simulink model "memristors_LSTM"  (R2020b)
settings: Solver=VariableStepAuto  StartTime=0.0  StopTime=3  RelTol=1e-3
libraries: simulink x17
(part 3 of 5)

== system memristors_LSTM/Subsystem/Memristor crossbar2/Subsystem2 ==
  note: Memristor
  note: k
  note: for I-V
  note: Rmem
  note: f(x)
  note: for x
  note: for processing
  In1 : Inport
  " V" : Sin  Frequency=0.5  SampleTime=0
  2p : Gain  Gain=2
  2x : Gain  Gain=2
  Add : Sum  Inputs=-+
  Add1 : Sum
  Add2 : Sum  Inputs=-+
  Add3 : Sum  Inputs=+-
  Add4 : Sum
  Constant : Constant
  Constant10 : Constant  Value=0
  Constant4 : Constant
  Constant9 : Constant
  D : Constant  Value=10^(-8)
  Divide : Product  Inputs=*/
  Divide1 : Product  Inputs=**/
  Gain2 : Gain  Gain=0.5
  I-t : Scope
  Integrator : Integrator
  Integrator Initial condition source : Integrator  InitialConditionSource=external
  Math Function : Math  Operator=pow  SaturateOnIntegerOverflow=on
  Math Function1 : Math  Operator=square  SaturateOnIntegerOverflow=on
  Product1 : Product
  Product2 : Product
  Product3 : Product  Inputs=3
  Product4 : Product
  R_off : Constant  Value=20000
  R_on : Constant  Value=100
  R_on1 : Constant  Value=100
  Switch : Switch  Threshold=1
  Switch1 : Switch
  V-t : Scope
  p : Constant  Value=10
  x-t : Scope
  x0 : Constant  Value=0.7
  𝜇_𝑣 : Constant  Value=10^(-14)
  Out1 : Outport
  Out2 : Outport  Port=2
  wires:
  Constant9/1 -> Switch/1
  Switch/1 -> Switch1/2, Switch1/1
  R_on/1 -> Divide1/1
  Integrator Initial condition source/1 -> Switch/3, Switch/2, x-t/1
  2p/1 -> Math Function/2
  Divide/1 -> I-t/1, Product3/1
  Switch1/1 -> Product2/2, Add/1, 2x/1
  𝜇_𝑣/1 -> Divide1/2
  Gain2/1 -> Integrator/1
  Math Function/1 -> Add3/2
  Add/1 -> Product1/1
  R_on1/1 -> Product2/1
  Constant/1 -> Add/2
  p/1 -> 2p/1
  D/1 -> Math Function1/1
  Divide1/1 -> Product3/3
  2x/1 -> Add2/2
  Product1/1 -> Add1/2
  R_off/1 -> Product1/2
  Add2/1 -> Math Function/1
  Constant4/1 -> Add3/1, Add2/1
  Product4/1 -> Out1/1, Out2/1, V-t/1
  Product2/1 -> Add1/1
  x0/1 -> Integrator Initial condition source/2
  Constant10/1 -> Switch1/3
  Product3/1 -> Integrator Initial condition source/1
  Add1/1 -> Divide/2
  Add3/1 -> Product3/2
  Math Function1/1 -> Divide1/3
  " V"/1 -> Add4/2
  In1/1 -> Add4/1
  Add4/1 -> Product4/1, Gain2/1
  Integrator/1 -> Divide/1, Product4/2

== system memristors_LSTM/Subsystem/Memristor crossbar2/Subsystem20 ==
  note: Memristor
  note: k
  note: for I-V
  note: Rmem
  note: f(x)
  note: for x
  note: for processing
  " V" : Sin  Amplitude=0.1  Frequency=0.5  SampleTime=0
  2p : Gain  Gain=2
  2x : Gain  Gain=2
  Add : Sum  Inputs=-+
  Add1 : Sum
  Add2 : Sum  Inputs=-+
  Add3 : Sum  Inputs=+-
  Constant : Constant
  Constant10 : Constant  Value=0
  Constant4 : Constant
  Constant9 : Constant
  D : Constant  Value=10^(-8)
  Divide : Product  Inputs=*/
  Divide1 : Product  Inputs=**/
  Gain2 : Gain  Gain=0.5
  I-t : Scope
  Integrator : Integrator
  Integrator Initial condition source : Integrator  InitialConditionSource=external
  Math Function : Math  Operator=pow  SaturateOnIntegerOverflow=on
  Math Function1 : Math  Operator=square  SaturateOnIntegerOverflow=on
  Product1 : Product
  Product2 : Product
  Product3 : Product  Inputs=3
  Product4 : Product
  R_off : Constant  Value=20000
  R_on : Constant  Value=100
  R_on1 : Constant  Value=100
  Switch : Switch  Threshold=1
  Switch1 : Switch
  V-t : Scope
  p : Constant  Value=10
  x-t : Scope
  x0 : Constant  Value=0.7
  𝜇_𝑣 : Constant  Value=10^(-14)
  Out1 : Outport
  Out2 : Outport  Port=2
  wires:
  Constant9/1 -> Switch/1
  Switch/1 -> Switch1/2, Switch1/1
  R_on/1 -> Divide1/1
  Integrator Initial condition source/1 -> Switch/3, Switch/2, x-t/1
  Integrator/1 -> Divide/1, Product4/2
  2p/1 -> Math Function/2
  Divide/1 -> I-t/1, Product3/1
  Switch1/1 -> Product2/2, Add/1, 2x/1
  𝜇_𝑣/1 -> Divide1/2
  Gain2/1 -> Integrator/1
  Math Function/1 -> Add3/2
  Add/1 -> Product1/1
  R_on1/1 -> Product2/1
  Constant/1 -> Add/2
  p/1 -> 2p/1
  D/1 -> Math Function1/1
  Divide1/1 -> Product3/3
  2x/1 -> Add2/2
  Product1/1 -> Add1/2
  R_off/1 -> Product1/2
  Add2/1 -> Math Function/1
  Constant4/1 -> Add3/1, Add2/1
  Product4/1 -> Out1/1, Out2/1, V-t/1
  Product2/1 -> Add1/1
  x0/1 -> Integrator Initial condition source/2
  Constant10/1 -> Switch1/3
  Product3/1 -> Integrator Initial condition source/1
  Add1/1 -> Divide/2
  Add3/1 -> Product3/2
  Math Function1/1 -> Divide1/3
  " V"/1 -> Gain2/1, Product4/1

== system memristors_LSTM/Subsystem/Memristor crossbar2/Subsystem21 ==
  note: Memristor
  note: k
  note: for I-V
  note: Rmem
  note: f(x)
  note: for x
  note: for processing
  In1 : Inport
  " V" : Sin  Amplitude=0.1  Frequency=0.5  SampleTime=0
  2p : Gain  Gain=2
  2x : Gain  Gain=2
  Add : Sum  Inputs=-+
  Add1 : Sum
  Add2 : Sum  Inputs=-+
  Add3 : Sum  Inputs=+-
  Add4 : Sum
  Constant : Constant
  Constant10 : Constant  Value=0
  Constant4 : Constant
  Constant9 : Constant
  D : Constant  Value=10^(-8)
  Divide : Product  Inputs=*/
  Divide1 : Product  Inputs=**/
  Gain2 : Gain  Gain=0.5
  I-t : Scope
  Integrator : Integrator
  Integrator Initial condition source : Integrator  InitialConditionSource=external
  Math Function : Math  Operator=pow  SaturateOnIntegerOverflow=on
  Math Function1 : Math  Operator=square  SaturateOnIntegerOverflow=on
  Product1 : Product
  Product2 : Product
  Product3 : Product  Inputs=3
  Product4 : Product
  R_off : Constant  Value=20000
  R_on : Constant  Value=100
  R_on1 : Constant  Value=100
  Switch : Switch  Threshold=1
  Switch1 : Switch
  V-t : Scope
  p : Constant  Value=10
  x-t : Scope
  x0 : Constant  Value=0.7
  𝜇_𝑣 : Constant  Value=10^(-14)
  Out1 : Outport
  Out2 : Outport  Port=2
  wires:
  Constant9/1 -> Switch/1
  Switch/1 -> Switch1/2, Switch1/1
  R_on/1 -> Divide1/1
  Integrator Initial condition source/1 -> Switch/3, Switch/2, x-t/1
  2p/1 -> Math Function/2
  Divide/1 -> I-t/1, Product3/1
  Switch1/1 -> Product2/2, Add/1, 2x/1
  𝜇_𝑣/1 -> Divide1/2
  Gain2/1 -> Integrator/1
  Math Function/1 -> Add3/2
  Add/1 -> Product1/1
  R_on1/1 -> Product2/1
  Constant/1 -> Add/2
  p/1 -> 2p/1
  D/1 -> Math Function1/1
  Divide1/1 -> Product3/3
  2x/1 -> Add2/2
  Product1/1 -> Add1/2
  R_off/1 -> Product1/2
  Add2/1 -> Math Function/1
  Constant4/1 -> Add3/1, Add2/1
  Product4/1 -> Out1/1, Out2/1, V-t/1
  Product2/1 -> Add1/1
  x0/1 -> Integrator Initial condition source/2
  Constant10/1 -> Switch1/3
  Product3/1 -> Integrator Initial condition source/1
  Add1/1 -> Divide/2
  Add3/1 -> Product3/2
  Math Function1/1 -> Divide1/3
  " V"/1 -> Add4/2
  In1/1 -> Add4/1
  Add4/1 -> Product4/1, Gain2/1
  Integrator/1 -> Divide/1, Product4/2

== system memristors_LSTM/Subsystem/Memristor crossbar2/Subsystem22 ==
  note: k
  note: for I-V
  note: Rmem
  note: f(x)
  note: for x
  note: for processing
  In1 : Inport
  " V" : Sin  Amplitude=0.1  Frequency=0.5  SampleTime=0
  2p : Gain  Gain=2
  2x : Gain  Gain=2
  Add : Sum  Inputs=-+
  Add1 : Sum
  Add2 : Sum  Inputs=-+
  Add3 : Sum  Inputs=+-
  Add4 : Sum
  Constant : Constant
  Constant10 : Constant  Value=0
  Constant4 : Constant
  Constant9 : Constant
  D : Constant  Value=10^(-8)
  Divide : Product  Inputs=*/
  Divide1 : Product  Inputs=**/
  Gain2 : Gain  Gain=0.5
  I-t : Scope
  Integrator : Integrator
  Integrator Initial condition source : Integrator  InitialConditionSource=external
  Math Function : Math  Operator=pow  SaturateOnIntegerOverflow=on
  Math Function1 : Math  Operator=square  SaturateOnIntegerOverflow=on
  Product1 : Product
  Product2 : Product
  Product3 : Product  Inputs=3
  Product4 : Product
  R_off : Constant  Value=20000
  R_on : Constant  Value=100
  R_on1 : Constant  Value=100
  Switch : Switch  Threshold=1
  Switch1 : Switch
  V-t : Scope
  p : Constant  Value=10
  x-t : Scope
  x0 : Constant  Value=0.7
  𝜇_𝑣 : Constant  Value=10^(-14)
  Out1 : Outport
  Out2 : Outport  Port=2
  wires:
  Constant9/1 -> Switch/1
  Switch/1 -> Switch1/2, Switch1/1
  R_on/1 -> Divide1/1
  Integrator Initial condition source/1 -> Switch/3, Switch/2, x-t/1
  Integrator/1 -> Divide/1, Product4/2
  2p/1 -> Math Function/2
  Divide/1 -> I-t/1, Product3/1
  Switch1/1 -> Product2/2, Add/1, 2x/1
  𝜇_𝑣/1 -> Divide1/2
  Gain2/1 -> Integrator/1
  Math Function/1 -> Add3/2
  Add/1 -> Product1/1
  R_on1/1 -> Product2/1
  Constant/1 -> Add/2
  p/1 -> 2p/1
  D/1 -> Math Function1/1
  Divide1/1 -> Product3/3
  2x/1 -> Add2/2
  Product1/1 -> Add1/2
  R_off/1 -> Product1/2
  Add2/1 -> Math Function/1
  Constant4/1 -> Add3/1, Add2/1
  Product2/1 -> Add1/1
  x0/1 -> Integrator Initial condition source/2
  Constant10/1 -> Switch1/3
  Product3/1 -> Integrator Initial condition source/1
  Add1/1 -> Divide/2
  Add3/1 -> Product3/2
  Math Function1/1 -> Divide1/3
  " V"/1 -> Add4/2
  In1/1 -> Add4/1
  Add4/1 -> Product4/1, Gain2/1
  Product4/1 -> Out1/1, Out2/1, V-t/1

== system memristors_LSTM/Subsystem/Memristor crossbar2/Subsystem23 ==
  note: Memristor
  note: k
  note: for I-V
  note: Rmem
  note: f(x)
  note: for x
  note: for processing
  In1 : Inport
  " V" : Sin  Amplitude=0.1  Frequency=0.5  SampleTime=0
  2p : Gain  Gain=2
  2x : Gain  Gain=2
  Add : Sum  Inputs=-+
  Add1 : Sum
  Add2 : Sum  Inputs=-+
  Add3 : Sum  Inputs=+-
  Add4 : Sum
  Constant : Constant
  Constant10 : Constant  Value=0
  Constant4 : Constant
  Constant9 : Constant
  D : Constant  Value=10^(-8)
  Divide : Product  Inputs=*/
  Divide1 : Product  Inputs=**/
  Gain2 : Gain  Gain=0.5
  I-t : Scope
  Integrator : Integrator
  Integrator Initial condition source : Integrator  InitialConditionSource=external
  Math Function : Math  Operator=pow  SaturateOnIntegerOverflow=on
  Math Function1 : Math  Operator=square  SaturateOnIntegerOverflow=on
  Product1 : Product
  Product2 : Product
  Product3 : Product  Inputs=3
  Product4 : Product
  R_off : Constant  Value=20000
  R_on : Constant  Value=100
  R_on1 : Constant  Value=100
  Switch : Switch  Threshold=1
  Switch1 : Switch
  V-t : Scope
  p : Constant  Value=10
  x-t : Scope
  x0 : Constant  Value=0.7
  𝜇_𝑣 : Constant  Value=10^(-14)
  Out1 : Outport
  Out2 : Outport  Port=2
  wires:
  Constant9/1 -> Switch/1
  Switch/1 -> Switch1/2, Switch1/1
  R_on/1 -> Divide1/1
  Integrator Initial condition source/1 -> Switch/3, Switch/2, x-t/1
  Integrator/1 -> Divide/1, Product4/2
  2p/1 -> Math Function/2
  Divide/1 -> I-t/1, Product3/1
  Switch1/1 -> Product2/2, Add/1, 2x/1
  𝜇_𝑣/1 -> Divide1/2
  Gain2/1 -> Integrator/1
  Math Function/1 -> Add3/2
  Add/1 -> Product1/1
  R_on1/1 -> Product2/1
  Constant/1 -> Add/2
  p/1 -> 2p/1
  D/1 -> Math Function1/1
  Divide1/1 -> Product3/3
  2x/1 -> Add2/2
  Product1/1 -> Add1/2
  R_off/1 -> Product1/2
  Add2/1 -> Math Function/1
  Constant4/1 -> Add3/1, Add2/1
  Product4/1 -> Out1/1, Out2/1, V-t/1
  Product2/1 -> Add1/1
  x0/1 -> Integrator Initial condition source/2
  Constant10/1 -> Switch1/3
  Product3/1 -> Integrator Initial condition source/1
  Add1/1 -> Divide/2
  Add3/1 -> Product3/2
  Math Function1/1 -> Divide1/3
  " V"/1 -> Add4/2
  In1/1 -> Add4/1
  Add4/1 -> Product4/1, Gain2/1

== system memristors_LSTM/Subsystem/Memristor crossbar2/Subsystem24 ==
  note: Memristor
  note: k
  note: for I-V
  note: Rmem
  note: f(x)
  note: for x
  note: for processing
  In1 : Inport
  " V" : Sin  Amplitude=0.1  Frequency=0.5  SampleTime=0
  2p : Gain  Gain=2
  2x : Gain  Gain=2
  Add : Sum  Inputs=-+
  Add1 : Sum
  Add2 : Sum  Inputs=-+
  Add3 : Sum  Inputs=+-
  Add4 : Sum
  Constant : Constant
  Constant10 : Constant  Value=0
  Constant4 : Constant
  Constant9 : Constant
  D : Constant  Value=10^(-8)
  Divide : Product  Inputs=*/
  Divide1 : Product  Inputs=**/
  Gain2 : Gain  Gain=0.5
  I-t : Scope
  Integrator : Integrator
  Integrator Initial condition source : Integrator  InitialConditionSource=external
  Math Function : Math  Operator=pow  SaturateOnIntegerOverflow=on
  Math Function1 : Math  Operator=square  SaturateOnIntegerOverflow=on
  Product1 : Product
  Product2 : Product
  Product3 : Product  Inputs=3
  Product4 : Product
  R_off : Constant  Value=20000
  R_on : Constant  Value=100
  R_on1 : Constant  Value=100
  Switch : Switch  Threshold=1
  Switch1 : Switch
  V-t : Scope
  XY Graph : simulink/Sinks/XY Graph  xmin=-1  xmax=1  ymin=-1  ymax=1  st=-1
  p : Constant  Value=10
  x-t : Scope
  x0 : Constant  Value=0.7
  𝜇_𝑣 : Constant  Value=10^(-14)
  Out2 : Outport
  wires:
  Constant9/1 -> Switch/1
  Switch/1 -> Switch1/2, Switch1/1
  R_on/1 -> Divide1/1
  Integrator Initial condition source/1 -> Switch/3, Switch/2, x-t/1
  Integrator/1 -> Divide/1, Product4/2
  2p/1 -> Math Function/2
  Divide/1 -> XY Graph/2, I-t/1, Product3/1
  Switch1/1 -> Product2/2, Add/1, 2x/1
  𝜇_𝑣/1 -> Divide1/2
  Gain2/1 -> Integrator/1
  Math Function/1 -> Add3/2
  Add/1 -> Product1/1
  R_on1/1 -> Product2/1
  Constant/1 -> Add/2
  p/1 -> 2p/1
  D/1 -> Math Function1/1
  Divide1/1 -> Product3/3
  2x/1 -> Add2/2
  Product1/1 -> Add1/2
  R_off/1 -> Product1/2
  Add2/1 -> Math Function/1
  Constant4/1 -> Add3/1, Add2/1
  Product2/1 -> Add1/1
  x0/1 -> Integrator Initial condition source/2
  Constant10/1 -> Switch1/3
  Product3/1 -> Integrator Initial condition source/1
  Add1/1 -> Divide/2
  Add3/1 -> Product3/2
  Math Function1/1 -> Divide1/3
  " V"/1 -> Add4/2
  In1/1 -> Add4/1
  Add4/1 -> Product4/1, Gain2/1
  Product4/1 -> XY Graph/1, Out2/1, V-t/1

== system memristors_LSTM/Subsystem/Memristor crossbar2/Subsystem25 ==
  note: k
  note: for I-V
  note: Rmem
  note: f(x)
  note: for x
  note: for processing
  In1 : Inport
  " V" : Sin  Frequency=0.5  SampleTime=0
  2p : Gain  Gain=2
  2x : Gain  Gain=2
  Add : Sum  Inputs=-+
  Add1 : Sum
  Add2 : Sum  Inputs=-+
  Add3 : Sum  Inputs=+-
  Add4 : Sum
  Constant : Constant
  Constant10 : Constant  Value=0
  Constant4 : Constant
  Constant9 : Constant
  D : Constant  Value=10^(-8)
  Divide : Product  Inputs=*/
  Divide1 : Product  Inputs=**/
  Gain2 : Gain  Gain=0.5
  I-t : Scope
  Integrator : Integrator
  Integrator Initial condition source : Integrator  InitialConditionSource=external
  Math Function : Math  Operator=pow  SaturateOnIntegerOverflow=on
  Math Function1 : Math  Operator=square  SaturateOnIntegerOverflow=on
  Product1 : Product
  Product2 : Product
  Product3 : Product  Inputs=3
  Product4 : Product
  R_off : Constant  Value=20000
  R_on : Constant  Value=100
  R_on1 : Constant  Value=100
  Switch : Switch  Threshold=1
  Switch1 : Switch
  V-t : Scope
  p : Constant  Value=10
  x-t : Scope
  x0 : Constant  Value=0.7
  𝜇_𝑣 : Constant  Value=10^(-14)
  Out1 : Outport
  Out2 : Outport  Port=2
  wires:
  Constant9/1 -> Switch/1
  Switch/1 -> Switch1/2, Switch1/1
  R_on/1 -> Divide1/1
  Integrator Initial condition source/1 -> Switch/3, Switch/2, x-t/1
  Integrator/1 -> Divide/1, Product4/2
  2p/1 -> Math Function/2
  Divide/1 -> I-t/1, Product3/1
  Switch1/1 -> Product2/2, Add/1, 2x/1
  𝜇_𝑣/1 -> Divide1/2
  Gain2/1 -> Integrator/1
  Math Function/1 -> Add3/2
  Add/1 -> Product1/1
  R_on1/1 -> Product2/1
  Constant/1 -> Add/2
  p/1 -> 2p/1
  D/1 -> Math Function1/1
  Divide1/1 -> Product3/3
  2x/1 -> Add2/2
  Product1/1 -> Add1/2
  R_off/1 -> Product1/2
  Add2/1 -> Math Function/1
  Constant4/1 -> Add3/1, Add2/1
  Product2/1 -> Add1/1
  x0/1 -> Integrator Initial condition source/2
  Constant10/1 -> Switch1/3
  Product3/1 -> Integrator Initial condition source/1
  Add1/1 -> Divide/2
  Add3/1 -> Product3/2
  Math Function1/1 -> Divide1/3
  " V"/1 -> Add4/2
  In1/1 -> Add4/1
  Add4/1 -> Product4/1, Gain2/1
  Product4/1 -> Out1/1, Out2/1, V-t/1

== system memristors_LSTM/Subsystem/Memristor crossbar2/Subsystem3 ==
  note: Memristor
  note: k
  note: for I-V
  note: Rmem
  note: f(x)
  note: for x
  note: for processing
  In1 : Inport
  " V" : Sin  Frequency=0.5  SampleTime=0
  2p : Gain  Gain=2
  2x : Gain  Gain=2
  Add : Sum  Inputs=-+
  Add1 : Sum
  Add2 : Sum  Inputs=-+
  Add3 : Sum  Inputs=+-
  Add4 : Sum
  Constant : Constant
  Constant10 : Constant  Value=0
  Constant4 : Constant
  Constant9 : Constant
  D : Constant  Value=10^(-8)
  Divide : Product  Inputs=*/
  Divide1 : Product  Inputs=**/
  Gain2 : Gain  Gain=0.5
  I-t : Scope
  Integrator : Integrator
  Integrator Initial condition source : Integrator  InitialConditionSource=external
  Math Function : Math  Operator=pow  SaturateOnIntegerOverflow=on
  Math Function1 : Math  Operator=square  SaturateOnIntegerOverflow=on
  Product1 : Product
  Product2 : Product
  Product3 : Product  Inputs=3
  Product4 : Product
  R_off : Constant  Value=20000
  R_on : Constant  Value=100
  R_on1 : Constant  Value=100
  Switch : Switch  Threshold=1
  Switch1 : Switch
  V-t : Scope
  p : Constant  Value=10
  x-t : Scope
  x0 : Constant  Value=0.7
  𝜇_𝑣 : Constant  Value=10^(-14)
  Out1 : Outport
  Out2 : Outport  Port=2
  wires:
  Constant9/1 -> Switch/1
  Switch/1 -> Switch1/2, Switch1/1
  R_on/1 -> Divide1/1
  Integrator Initial condition source/1 -> Switch/3, Switch/2, x-t/1
  Integrator/1 -> Divide/1, Product4/2
  2p/1 -> Math Function/2
  Divide/1 -> I-t/1, Product3/1
  Switch1/1 -> Product2/2, Add/1, 2x/1
  𝜇_𝑣/1 -> Divide1/2
  Gain2/1 -> Integrator/1
  Math Function/1 -> Add3/2
  Add/1 -> Product1/1
  R_on1/1 -> Product2/1
  Constant/1 -> Add/2
  p/1 -> 2p/1
  D/1 -> Math Function1/1
  Divide1/1 -> Product3/3
  2x/1 -> Add2/2
  Product1/1 -> Add1/2
  R_off/1 -> Product1/2
  Add2/1 -> Math Function/1
  Constant4/1 -> Add3/1, Add2/1
  Product4/1 -> Out1/1, Out2/1, V-t/1
  Product2/1 -> Add1/1
  x0/1 -> Integrator Initial condition source/2
  Constant10/1 -> Switch1/3
  Product3/1 -> Integrator Initial condition source/1
  Add1/1 -> Divide/2
  Add3/1 -> Product3/2
  Math Function1/1 -> Divide1/3
  " V"/1 -> Add4/2
  In1/1 -> Add4/1
  Add4/1 -> Product4/1, Gain2/1

== system memristors_LSTM/Subsystem/Memristor crossbar2/Subsystem4 ==
  note: Memristor
  note: k
  note: for I-V
  note: Rmem
  note: f(x)
  note: for x
  note: for processing
  In1 : Inport
  " V" : Sin  Frequency=0.5  SampleTime=0
  2p : Gain  Gain=2
  2x : Gain  Gain=2
  Add : Sum  Inputs=-+
  Add1 : Sum
  Add2 : Sum  Inputs=-+
  Add3 : Sum  Inputs=+-
  Add4 : Sum
  Constant : Constant
  Constant10 : Constant  Value=0
  Constant4 : Constant
  Constant9 : Constant
  D : Constant  Value=10^(-8)
  Divide : Product  Inputs=*/
  Divide1 : Product  Inputs=**/
  Gain2 : Gain  Gain=0.5
  I-t : Scope
  Integrator : Integrator
  Integrator Initial condition source : Integrator  InitialConditionSource=external
  Math Function : Math  Operator=pow  SaturateOnIntegerOverflow=on
  Math Function1 : Math  Operator=square  SaturateOnIntegerOverflow=on
  Product1 : Product
  Product2 : Product
  Product3 : Product  Inputs=3
  Product4 : Product
  R_off : Constant  Value=20000
  R_on : Constant  Value=100
  R_on1 : Constant  Value=100
  Switch : Switch  Threshold=1
  Switch1 : Switch
  V-t : Scope
  p : Constant  Value=10
  x-t : Scope
  x0 : Constant  Value=0.7
  𝜇_𝑣 : Constant  Value=10^(-14)
  Out2 : Outport
  wires:
  Constant9/1 -> Switch/1
  Switch/1 -> Switch1/2, Switch1/1
  R_on/1 -> Divide1/1
  Integrator Initial condition source/1 -> Switch/3, Switch/2, x-t/1
  Integrator/1 -> Divide/1, Product4/2
  2p/1 -> Math Function/2
  Divide/1 -> I-t/1, Product3/1
  Switch1/1 -> Product2/2, Add/1, 2x/1
  𝜇_𝑣/1 -> Divide1/2
  Gain2/1 -> Integrator/1
  Math Function/1 -> Add3/2
  Add/1 -> Product1/1
  R_on1/1 -> Product2/1
  Constant/1 -> Add/2
  p/1 -> 2p/1
  D/1 -> Math Function1/1
  Divide1/1 -> Product3/3
  2x/1 -> Add2/2
  Product1/1 -> Add1/2
  R_off/1 -> Product1/2
  Add2/1 -> Math Function/1
  Constant4/1 -> Add3/1, Add2/1
  Product4/1 -> Out2/1, V-t/1
  Product2/1 -> Add1/1
  x0/1 -> Integrator Initial condition source/2
  Constant10/1 -> Switch1/3
  Product3/1 -> Integrator Initial condition source/1
  Add1/1 -> Divide/2
  Add3/1 -> Product3/2
  Math Function1/1 -> Divide1/3
  " V"/1 -> Add4/2
  In1/1 -> Add4/1
  Add4/1 -> Product4/1, Gain2/1

== system memristors_LSTM/Subsystem/Memristor crossbar2/Subsystem5 ==
  note: Memristor
  note: k
  note: for I-V
  note: Rmem
  note: f(x)
  note: for x
  note: for processing
  " V" : Sin  Amplitude=0.1  Frequency=0.5  SampleTime=0
  2p : Gain  Gain=2
  2x : Gain  Gain=2
  Add : Sum  Inputs=-+
  Add1 : Sum
  Add2 : Sum  Inputs=-+
  Add3 : Sum  Inputs=+-
  Constant : Constant
  Constant10 : Constant  Value=0
  Constant4 : Constant
  Constant9 : Constant
  D : Constant  Value=10^(-8)
  Divide : Product  Inputs=*/
  Divide1 : Product  Inputs=**/
  Gain2 : Gain  Gain=0.5
  I-t : Scope
  Integrator : Integrator
  Integrator Initial condition source : Integrator  InitialConditionSource=external
  Math Function : Math  Operator=pow  SaturateOnIntegerOverflow=on
  Math Function1 : Math  Operator=square  SaturateOnIntegerOverflow=on
  Product1 : Product
  Product2 : Product
  Product3 : Product  Inputs=3
  Product4 : Product
  R_off : Constant  Value=20000
  R_on : Constant  Value=100
  R_on1 : Constant  Value=100
  Switch : Switch  Threshold=1
  Switch1 : Switch
  V-t : Scope
  p : Constant  Value=10
  x-t : Scope
  x0 : Constant  Value=0.7
  𝜇_𝑣 : Constant  Value=10^(-14)
  Out1 : Outport
  Out2 : Outport  Port=2
  wires:
  Constant9/1 -> Switch/1
  Switch/1 -> Switch1/2, Switch1/1
  R_on/1 -> Divide1/1
  Integrator Initial condition source/1 -> Switch/3, Switch/2, x-t/1
  Integrator/1 -> Divide/1, Product4/2
  2p/1 -> Math Function/2
  Divide/1 -> I-t/1, Product3/1
  Switch1/1 -> Product2/2, Add/1, 2x/1
  𝜇_𝑣/1 -> Divide1/2
  Gain2/1 -> Integrator/1
  Math Function/1 -> Add3/2
  Add/1 -> Product1/1
  R_on1/1 -> Product2/1
  Constant/1 -> Add/2
  p/1 -> 2p/1
  D/1 -> Math Function1/1
  Divide1/1 -> Product3/3
  2x/1 -> Add2/2
  Product1/1 -> Add1/2
  R_off/1 -> Product1/2
  Add2/1 -> Math Function/1
  Constant4/1 -> Add3/1, Add2/1
  Product4/1 -> Out1/1, Out2/1, V-t/1
  Product2/1 -> Add1/1
  x0/1 -> Integrator Initial condition source/2
  Constant10/1 -> Switch1/3
  Product3/1 -> Integrator Initial condition source/1
  Add1/1 -> Divide/2
  Add3/1 -> Product3/2
  Math Function1/1 -> Divide1/3
  " V"/1 -> Gain2/1, Product4/1

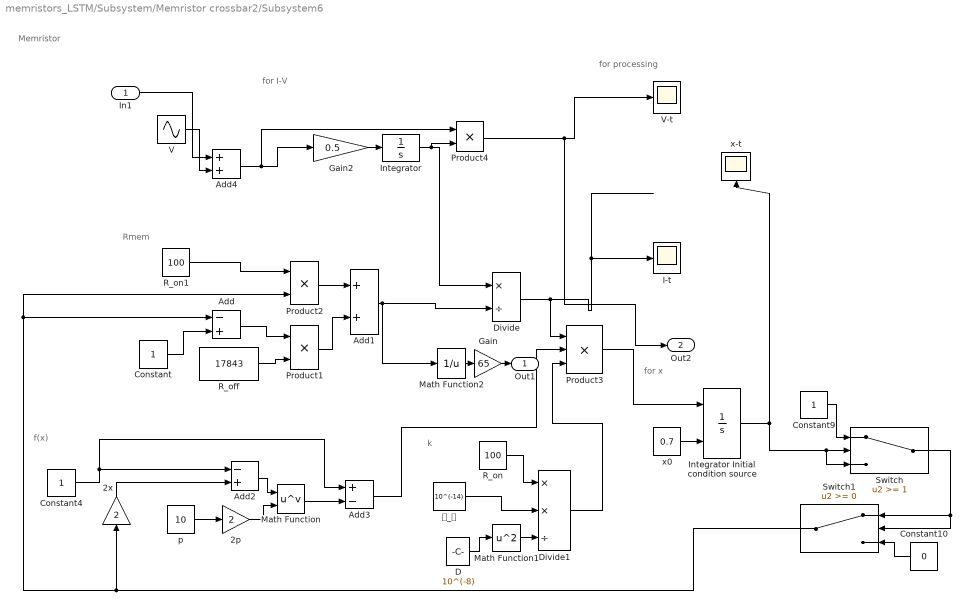
== system memristors_LSTM/Subsystem/Memristor crossbar2/Subsystem6 ==
  note: Memristor
  note: k
  note: for I-V
  note: Rmem
  note: f(x)
  note: for x
  note: for processing
  In1 : Inport
  " V" : Sin  Frequency=0.5  SampleTime=0
  2p : Gain  Gain=2
  2x : Gain  Gain=2
  Add : Sum  Inputs=-+
  Add1 : Sum
  Add2 : Sum  Inputs=-+
  Add3 : Sum  Inputs=+-
  Add4 : Sum
  Constant : Constant
  Constant10 : Constant  Value=0
  Constant4 : Constant
  Constant9 : Constant
  D : Constant  Value=10^(-8)
  Divide : Product  Inputs=*/
  Divide1 : Product  Inputs=**/
  Gain : Gain  Gain=65
  Gain2 : Gain  Gain=0.5
  I-t : Scope
  Integrator : Integrator
  Integrator Initial condition source : Integrator  InitialConditionSource=external
  Math Function : Math  Operator=pow  SaturateOnIntegerOverflow=on
  Math Function1 : Math  Operator=square  SaturateOnIntegerOverflow=on
  Math Function2 : Math  Operator=reciprocal  SaturateOnIntegerOverflow=on
  Product1 : Product
  Product2 : Product
  Product3 : Product  Inputs=3
  Product4 : Product
  R_off : Constant  Value=17843
  R_on : Constant  Value=100
  R_on1 : Constant  Value=100
  Switch : Switch  Threshold=1
  Switch1 : Switch
  V-t : Scope
  p : Constant  Value=10
  x-t : Scope
  x0 : Constant  Value=0.7
  𝜇_𝑣 : Constant  Value=10^(-14)
  Out1 : Outport
  Out2 : Outport  Port=2
  wires:
  Constant9/1 -> Switch/1
  Switch/1 -> Switch1/2, Switch1/1
  R_on/1 -> Divide1/1
  Integrator Initial condition source/1 -> Switch/3, Switch/2, x-t/1
  2p/1 -> Math Function/2
  Divide/1 -> I-t/1, Product3/1
  Switch1/1 -> Product2/2, Add/1, 2x/1
  𝜇_𝑣/1 -> Divide1/2
  Gain2/1 -> Integrator/1
  Math Function/1 -> Add3/2
  Add/1 -> Product1/1
  R_on1/1 -> Product2/1
  Constant/1 -> Add/2
  p/1 -> 2p/1
  D/1 -> Math Function1/1
  Divide1/1 -> Product3/3
  2x/1 -> Add2/2
  Product1/1 -> Add1/2
  R_off/1 -> Product1/2
  Add2/1 -> Math Function/1
  Constant4/1 -> Add3/1, Add2/1
  Product4/1 -> Out2/1, V-t/1
  Product2/1 -> Add1/1
  x0/1 -> Integrator Initial condition source/2
  Constant10/1 -> Switch1/3
  Product3/1 -> Integrator Initial condition source/1
  Add3/1 -> Product3/2
  Math Function1/1 -> Divide1/3
  " V"/1 -> Add4/2
  In1/1 -> Add4/1
  Add4/1 -> Product4/1, Gain2/1
  Integrator/1 -> Divide/1, Product4/2
  Add1/1 -> Math Function2/1, Divide/2
  Math Function2/1 -> Gain/1
  Gain/1 -> Out1/1

== system memristors_LSTM/Subsystem/Memristor crossbar2/Subsystem7 ==
  note: k
  note: for I-V
  note: Rmem
  note: f(x)
  note: for x
  note: for processing
  In1 : Inport
  " V" : Sin  Frequency=0.5  SampleTime=0
  2p : Gain  Gain=2
  2x : Gain  Gain=2
  Add : Sum  Inputs=-+
  Add1 : Sum
  Add2 : Sum  Inputs=-+
  Add3 : Sum  Inputs=+-
  Add4 : Sum
  Constant : Constant
  Constant10 : Constant  Value=0
  Constant4 : Constant
  Constant9 : Constant
  D : Constant  Value=10^(-8)
  Divide : Product  Inputs=*/
  Divide1 : Product  Inputs=**/
  Gain2 : Gain  Gain=0.5
  I-t : Scope
  Integrator : Integrator
  Integrator Initial condition source : Integrator  InitialConditionSource=external
  Math Function : Math  Operator=pow  SaturateOnIntegerOverflow=on
  Math Function1 : Math  Operator=square  SaturateOnIntegerOverflow=on
  Product1 : Product
  Product2 : Product
  Product3 : Product  Inputs=3
  Product4 : Product
  R_off : Constant  Value=20000
  R_on : Constant  Value=100
  R_on1 : Constant  Value=100
  Switch : Switch  Threshold=1
  Switch1 : Switch
  V-t : Scope
  p : Constant  Value=10
  x-t : Scope
  x0 : Constant  Value=0.7
  𝜇_𝑣 : Constant  Value=10^(-14)
  Out1 : Outport
  Out2 : Outport  Port=2
  wires:
  Constant9/1 -> Switch/1
  Switch/1 -> Switch1/2, Switch1/1
  R_on/1 -> Divide1/1
  Integrator Initial condition source/1 -> Switch/3, Switch/2, x-t/1
  Integrator/1 -> Divide/1, Product4/2
  2p/1 -> Math Function/2
  Divide/1 -> I-t/1, Product3/1
  Switch1/1 -> Product2/2, Add/1, 2x/1
  𝜇_𝑣/1 -> Divide1/2
  Gain2/1 -> Integrator/1
  Math Function/1 -> Add3/2
  Add/1 -> Product1/1
  R_on1/1 -> Product2/1
  Constant/1 -> Add/2
  p/1 -> 2p/1
  D/1 -> Math Function1/1
  Divide1/1 -> Product3/3
  2x/1 -> Add2/2
  Product1/1 -> Add1/2
  R_off/1 -> Product1/2
  Add2/1 -> Math Function/1
  Constant4/1 -> Add3/1, Add2/1
  Product2/1 -> Add1/1
  x0/1 -> Integrator Initial condition source/2
  Constant10/1 -> Switch1/3
  Product3/1 -> Integrator Initial condition source/1
  Add1/1 -> Divide/2
  Add3/1 -> Product3/2
  Math Function1/1 -> Divide1/3
  " V"/1 -> Add4/2
  In1/1 -> Add4/1
  Add4/1 -> Product4/1, Gain2/1
  Product4/1 -> Out1/1, Out2/1, V-t/1

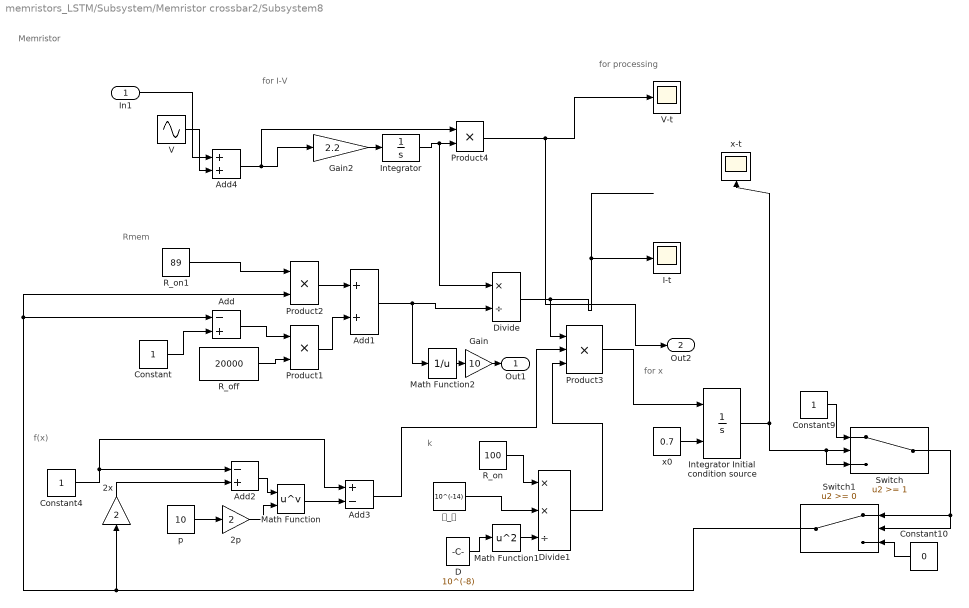
== system memristors_LSTM/Subsystem/Memristor crossbar2/Subsystem8 ==
  note: Memristor
  note: k
  note: for I-V
  note: Rmem
  note: f(x)
  note: for x
  note: for processing
  In1 : Inport
  " V" : Sin  Frequency=0.5  SampleTime=0
  2p : Gain  Gain=2
  2x : Gain  Gain=2
  Add : Sum  Inputs=-+
  Add1 : Sum
  Add2 : Sum  Inputs=-+
  Add3 : Sum  Inputs=+-
  Add4 : Sum
  Constant : Constant
  Constant10 : Constant  Value=0
  Constant4 : Constant
  Constant9 : Constant
  D : Constant  Value=10^(-8)
  Divide : Product  Inputs=*/
  Divide1 : Product  Inputs=**/
  Gain : Gain  Gain=10
  Gain2 : Gain  Gain=2.2
  I-t : Scope
  Integrator : Integrator
  Integrator Initial condition source : Integrator  InitialConditionSource=external
  Math Function : Math  Operator=pow  SaturateOnIntegerOverflow=on
  Math Function1 : Math  Operator=square  SaturateOnIntegerOverflow=on
  Math Function2 : Math  Operator=reciprocal  SaturateOnIntegerOverflow=on
  Product1 : Product
  Product2 : Product
  Product3 : Product  Inputs=3
  Product4 : Product
  R_off : Constant  Value=20000
  R_on : Constant  Value=100
  R_on1 : Constant  Value=89
  Switch : Switch  Threshold=1
  Switch1 : Switch
  V-t : Scope
  p : Constant  Value=10
  x-t : Scope
  x0 : Constant  Value=0.7
  𝜇_𝑣 : Constant  Value=10^(-14)
  Out1 : Outport
  Out2 : Outport  Port=2
  wires:
  Constant9/1 -> Switch/1
  Switch/1 -> Switch1/2, Switch1/1
  R_on/1 -> Divide1/1
  Integrator Initial condition source/1 -> Switch/3, Switch/2, x-t/1
  Integrator/1 -> Divide/1, Product4/2
  2p/1 -> Math Function/2
  Divide/1 -> I-t/1, Product3/1
  Switch1/1 -> Product2/2, Add/1, 2x/1
  𝜇_𝑣/1 -> Divide1/2
  Gain2/1 -> Integrator/1
  Math Function/1 -> Add3/2
  Add/1 -> Product1/1
  R_on1/1 -> Product2/1
  Constant/1 -> Add/2
  p/1 -> 2p/1
  D/1 -> Math Function1/1
  Divide1/1 -> Product3/3
  2x/1 -> Add2/2
  Product1/1 -> Add1/2
  R_off/1 -> Product1/2
  Add2/1 -> Math Function/1
  Constant4/1 -> Add3/1, Add2/1
  Product4/1 -> Out2/1, V-t/1
  Product2/1 -> Add1/1
  x0/1 -> Integrator Initial condition source/2
  Constant10/1 -> Switch1/3
  Product3/1 -> Integrator Initial condition source/1
  Add3/1 -> Product3/2
  Math Function1/1 -> Divide1/3
  " V"/1 -> Add4/2
  In1/1 -> Add4/1
  Add4/1 -> Product4/1, Gain2/1
  Add1/1 -> Math Function2/1, Divide/2
  Math Function2/1 -> Gain/1
  Gain/1 -> Out1/1

== system memristors_LSTM/Subsystem/Memristor crossbar2/Subsystem9 ==
  note: Memristor
  note: k
  note: for I-V
  note: Rmem
  note: f(x)
  note: for x
  note: for processing
  In1 : Inport
  " V" : Sin  Frequency=0.5  SampleTime=0
  2p : Gain  Gain=2
  2x : Gain  Gain=2
  Add : Sum  Inputs=-+
  Add1 : Sum
  Add2 : Sum  Inputs=-+
  Add3 : Sum  Inputs=+-
  Add4 : Sum
  Constant : Constant
  Constant10 : Constant  Value=0
  Constant4 : Constant
  Constant9 : Constant
  D : Constant  Value=10^(-8)
  Divide : Product  Inputs=*/
  Divide1 : Product  Inputs=**/
  Gain2 : Gain  Gain=0.5
  I-t : Scope
  Integrator : Integrator
  Integrator Initial condition source : Integrator  InitialConditionSource=external
  Math Function : Math  Operator=pow  SaturateOnIntegerOverflow=on
  Math Function1 : Math  Operator=square  SaturateOnIntegerOverflow=on
  Product1 : Product
  Product2 : Product
  Product3 : Product  Inputs=3
  Product4 : Product
  R_off : Constant  Value=20000
  R_on : Constant  Value=100
  R_on1 : Constant  Value=100
  Switch : Switch  Threshold=1
  Switch1 : Switch
  V-t : Scope
  p : Constant  Value=10
  x-t : Scope
  x0 : Constant  Value=0.7
  𝜇_𝑣 : Constant  Value=10^(-14)
  Out2 : Outport
  wires:
  Constant9/1 -> Switch/1
  Switch/1 -> Switch1/2, Switch1/1
  R_on/1 -> Divide1/1
  Integrator Initial condition source/1 -> Switch/3, Switch/2, x-t/1
  Integrator/1 -> Divide/1, Product4/2
  2p/1 -> Math Function/2
  Divide/1 -> I-t/1, Product3/1
  Switch1/1 -> Product2/2, Add/1, 2x/1
  𝜇_𝑣/1 -> Divide1/2
  Gain2/1 -> Integrator/1
  Math Function/1 -> Add3/2
  Add/1 -> Product1/1
  R_on1/1 -> Product2/1
  Constant/1 -> Add/2
  p/1 -> 2p/1
  D/1 -> Math Function1/1
  Divide1/1 -> Product3/3
  2x/1 -> Add2/2
  Product1/1 -> Add1/2
  R_off/1 -> Product1/2
  Add2/1 -> Math Function/1
  Constant4/1 -> Add3/1, Add2/1
  Product4/1 -> Out2/1, V-t/1
  Product2/1 -> Add1/1
  x0/1 -> Integrator Initial condition source/2
  Constant10/1 -> Switch1/3
  Product3/1 -> Integrator Initial condition source/1
  Add1/1 -> Divide/2
  Add3/1 -> Product3/2
  Math Function1/1 -> Divide1/3
  " V"/1 -> Add4/2
  In1/1 -> Add4/1
  Add4/1 -> Product4/1, Gain2/1

== system memristors_LSTM/Subsystem/Memristor crossbar4/Subsystem1 ==
  note: Memristor
  note: k
  note: for I-V
  note: Rmem
  note: f(x)
  note: for x
  note: for processing
  " V" : Sin  Amplitude=0.1  Frequency=0.5  SampleTime=0
  2p : Gain  Gain=2
  2x : Gain  Gain=2
  Add : Sum  Inputs=-+
  Add1 : Sum
  Add2 : Sum  Inputs=-+
  Add3 : Sum  Inputs=+-
  Constant : Constant
  Constant10 : Constant  Value=0
  Constant4 : Constant
  Constant9 : Constant
  D : Constant  Value=10^(-8)
  Divide : Product  Inputs=*/
  Divide1 : Product  Inputs=**/
  Gain2 : Gain  Gain=0.5
  I-t : Scope
  Integrator : Integrator
  Integrator Initial condition source : Integrator  InitialConditionSource=external
  Math Function : Math  Operator=pow  SaturateOnIntegerOverflow=on
  Math Function1 : Math  Operator=square  SaturateOnIntegerOverflow=on
  Product1 : Product
  Product2 : Product
  Product3 : Product  Inputs=3
  Product4 : Product
  R_off : Constant  Value=20000
  R_on : Constant  Value=100
  R_on1 : Constant  Value=100
  Switch : Switch  Threshold=1
  Switch1 : Switch
  V-t : Scope
  XY Graph : simulink/Sinks/XY Graph  xmin=-0.05  xmax=0.05  ymin=-0.01  ymax=0.01  st=-1
  p : Constant  Value=10
  x-t : Scope
  x0 : Constant  Value=0.7
  𝜇_𝑣 : Constant  Value=10^(-14)
  Out1 : Outport
  Out2 : Outport  Port=2
  wires:
  Constant9/1 -> Switch/1
  Switch/1 -> Switch1/2, Switch1/1
  R_on/1 -> Divide1/1
  Integrator Initial condition source/1 -> Switch/3, Switch/2, x-t/1
  Integrator/1 -> Divide/1, Product4/2
  2p/1 -> Math Function/2
  Divide/1 -> XY Graph/2, I-t/1, Product3/1
  Switch1/1 -> Product2/2, Add/1, 2x/1
  𝜇_𝑣/1 -> Divide1/2
  Gain2/1 -> Integrator/1
  Math Function/1 -> Add3/2
  Add/1 -> Product1/1
  R_on1/1 -> Product2/1
  Constant/1 -> Add/2
  p/1 -> 2p/1
  D/1 -> Math Function1/1
  Divide1/1 -> Product3/3
  2x/1 -> Add2/2
  Product1/1 -> Add1/2
  R_off/1 -> Product1/2
  Add2/1 -> Math Function/1
  Constant4/1 -> Add3/1, Add2/1
  Product4/1 -> Out1/1, XY Graph/1, Out2/1, V-t/1
  Product2/1 -> Add1/1
  x0/1 -> Integrator Initial condition source/2
  Constant10/1 -> Switch1/3
  Product3/1 -> Integrator Initial condition source/1
  Add1/1 -> Divide/2
  Add3/1 -> Product3/2
  Math Function1/1 -> Divide1/3
  " V"/1 -> Gain2/1, Product4/1

== system memristors_LSTM/Subsystem/Memristor crossbar4/Subsystem10 ==
  note: Memristor
  note: k
  note: for I-V
  note: Rmem
  note: f(x)
  note: for x
  note: for processing
  " V" : Sin  Amplitude=0.1  Frequency=0.5  SampleTime=0
  2p : Gain  Gain=2
  2x : Gain  Gain=2
  Add : Sum  Inputs=-+
  Add1 : Sum
  Add2 : Sum  Inputs=-+
  Add3 : Sum  Inputs=+-
  Constant : Constant
  Constant10 : Constant  Value=0
  Constant4 : Constant
  Constant9 : Constant
  D : Constant  Value=10^(-8)
  Divide : Product  Inputs=*/
  Divide1 : Product  Inputs=**/
  Gain2 : Gain  Gain=0.5
  I-t : Scope
  Integrator : Integrator
  Integrator Initial condition source : Integrator  InitialConditionSource=external
  Math Function : Math  Operator=pow  SaturateOnIntegerOverflow=on
  Math Function1 : Math  Operator=square  SaturateOnIntegerOverflow=on
  Product1 : Product
  Product2 : Product
  Product3 : Product  Inputs=3
  Product4 : Product
  R_off : Constant  Value=20000
  R_on : Constant  Value=100
  R_on1 : Constant  Value=100
  Switch : Switch  Threshold=1
  Switch1 : Switch
  V-t : Scope
  p : Constant  Value=10
  x-t : Scope
  x0 : Constant  Value=0.7
  𝜇_𝑣 : Constant  Value=10^(-14)
  Out1 : Outport
  Out2 : Outport  Port=2
  wires:
  Constant9/1 -> Switch/1
  Switch/1 -> Switch1/2, Switch1/1
  R_on/1 -> Divide1/1
  Integrator Initial condition source/1 -> Switch/3, Switch/2, x-t/1
  Integrator/1 -> Divide/1, Product4/2
  2p/1 -> Math Function/2
  Divide/1 -> I-t/1, Product3/1
  Switch1/1 -> Product2/2, Add/1, 2x/1
  𝜇_𝑣/1 -> Divide1/2
  Gain2/1 -> Integrator/1
  Math Function/1 -> Add3/2
  Add/1 -> Product1/1
  R_on1/1 -> Product2/1
  Constant/1 -> Add/2
  p/1 -> 2p/1
  D/1 -> Math Function1/1
  Divide1/1 -> Product3/3
  2x/1 -> Add2/2
  Product1/1 -> Add1/2
  R_off/1 -> Product1/2
  Add2/1 -> Math Function/1
  Constant4/1 -> Add3/1, Add2/1
  Product4/1 -> Out1/1, Out2/1, V-t/1
  Product2/1 -> Add1/1
  x0/1 -> Integrator Initial condition source/2
  Constant10/1 -> Switch1/3
  Product3/1 -> Integrator Initial condition source/1
  Add1/1 -> Divide/2
  Add3/1 -> Product3/2
  Math Function1/1 -> Divide1/3
  " V"/1 -> Gain2/1, Product4/1

== system memristors_LSTM/Subsystem/Memristor crossbar4/Subsystem11 ==
  note: Memristor
  note: k
  note: for I-V
  note: Rmem
  note: f(x)
  note: for x
  note: for processing
  In1 : Inport
  " V" : Sin  Frequency=0.5  SampleTime=0
  2p : Gain  Gain=2
  2x : Gain  Gain=2
  Add : Sum  Inputs=-+
  Add1 : Sum
  Add2 : Sum  Inputs=-+
  Add3 : Sum  Inputs=+-
  Add4 : Sum
  Constant : Constant
  Constant10 : Constant  Value=0
  Constant4 : Constant
  Constant9 : Constant
  D : Constant  Value=10^(-8)
  Divide : Product  Inputs=*/
  Divide1 : Product  Inputs=**/
  Gain2 : Gain  Gain=0.5
  I-t : Scope
  Integrator : Integrator
  Integrator Initial condition source : Integrator  InitialConditionSource=external
  Math Function : Math  Operator=pow  SaturateOnIntegerOverflow=on
  Math Function1 : Math  Operator=square  SaturateOnIntegerOverflow=on
  Product1 : Product
  Product2 : Product
  Product3 : Product  Inputs=3
  Product4 : Product
  R_off : Constant  Value=20000
  R_on : Constant  Value=100
  R_on1 : Constant  Value=100
  Switch : Switch  Threshold=1
  Switch1 : Switch
  V-t : Scope
  p : Constant  Value=10
  x-t : Scope
  x0 : Constant  Value=0.7
  𝜇_𝑣 : Constant  Value=10^(-14)
  Out1 : Outport
  Out2 : Outport  Port=2
  wires:
  Constant9/1 -> Switch/1
  Switch/1 -> Switch1/2, Switch1/1
  R_on/1 -> Divide1/1
  Integrator Initial condition source/1 -> Switch/3, Switch/2, x-t/1
  2p/1 -> Math Function/2
  Divide/1 -> I-t/1, Product3/1
  Switch1/1 -> Product2/2, Add/1, 2x/1
  𝜇_𝑣/1 -> Divide1/2
  Gain2/1 -> Integrator/1
  Math Function/1 -> Add3/2
  Add/1 -> Product1/1
  R_on1/1 -> Product2/1
  Constant/1 -> Add/2
  p/1 -> 2p/1
  D/1 -> Math Function1/1
  Divide1/1 -> Product3/3
  2x/1 -> Add2/2
  Product1/1 -> Add1/2
  R_off/1 -> Product1/2
  Add2/1 -> Math Function/1
  Constant4/1 -> Add3/1, Add2/1
  Product4/1 -> Out1/1, Out2/1, V-t/1
  Product2/1 -> Add1/1
  x0/1 -> Integrator Initial condition source/2
  Constant10/1 -> Switch1/3
  Product3/1 -> Integrator Initial condition source/1
  Add1/1 -> Divide/2
  Add3/1 -> Product3/2
  Math Function1/1 -> Divide1/3
  " V"/1 -> Add4/2
  In1/1 -> Add4/1
  Add4/1 -> Product4/1, Gain2/1
  Integrator/1 -> Divide/1, Product4/2

== system memristors_LSTM/Subsystem/Memristor crossbar4/Subsystem12 ==
  note: k
  note: for I-V
  note: Rmem
  note: f(x)
  note: for x
  note: for processing
  In1 : Inport
  " V" : Sin  Frequency=0.5  SampleTime=0
  2p : Gain  Gain=2
  2x : Gain  Gain=2
  Add : Sum  Inputs=-+
  Add1 : Sum
  Add2 : Sum  Inputs=-+
  Add3 : Sum  Inputs=+-
  Add4 : Sum
  Constant : Constant
  Constant10 : Constant  Value=0
  Constant4 : Constant
  Constant9 : Constant
  D : Constant  Value=10^(-8)
  Divide : Product  Inputs=*/
  Divide1 : Product  Inputs=**/
  Gain2 : Gain  Gain=0.5
  I-t : Scope
  Integrator : Integrator
  Integrator Initial condition source : Integrator  InitialConditionSource=external
  Math Function : Math  Operator=pow  SaturateOnIntegerOverflow=on
  Math Function1 : Math  Operator=square  SaturateOnIntegerOverflow=on
  Product1 : Product
  Product2 : Product
  Product3 : Product  Inputs=3
  Product4 : Product
  R_off : Constant  Value=20000
  R_on : Constant  Value=100
  R_on1 : Constant  Value=100
  Switch : Switch  Threshold=1
  Switch1 : Switch
  V-t : Scope
  p : Constant  Value=10
  x-t : Scope
  x0 : Constant  Value=0.7
  𝜇_𝑣 : Constant  Value=10^(-14)
  Out1 : Outport
  Out2 : Outport  Port=2
  wires:
  Constant9/1 -> Switch/1
  Switch/1 -> Switch1/2, Switch1/1
  R_on/1 -> Divide1/1
  Integrator Initial condition source/1 -> Switch/3, Switch/2, x-t/1
  Integrator/1 -> Divide/1, Product4/2
  2p/1 -> Math Function/2
  Divide/1 -> I-t/1, Product3/1
  Switch1/1 -> Product2/2, Add/1, 2x/1
  𝜇_𝑣/1 -> Divide1/2
  Gain2/1 -> Integrator/1
  Math Function/1 -> Add3/2
  Add/1 -> Product1/1
  R_on1/1 -> Product2/1
  Constant/1 -> Add/2
  p/1 -> 2p/1
  D/1 -> Math Function1/1
  Divide1/1 -> Product3/3
  2x/1 -> Add2/2
  Product1/1 -> Add1/2
  R_off/1 -> Product1/2
  Add2/1 -> Math Function/1
  Constant4/1 -> Add3/1, Add2/1
  Product2/1 -> Add1/1
  x0/1 -> Integrator Initial condition source/2
  Constant10/1 -> Switch1/3
  Product3/1 -> Integrator Initial condition source/1
  Add1/1 -> Divide/2
  Add3/1 -> Product3/2
  Math Function1/1 -> Divide1/3
  " V"/1 -> Add4/2
  In1/1 -> Add4/1
  Add4/1 -> Product4/1, Gain2/1
  Product4/1 -> Out1/1, Out2/1, V-t/1

== system memristors_LSTM/Subsystem/Memristor crossbar4/Subsystem13 ==
  note: Memristor
  note: k
  note: for I-V
  note: Rmem
  note: f(x)
  note: for x
  note: for processing
  In1 : Inport
  " V" : Sin  Frequency=0.5  SampleTime=0
  2p : Gain  Gain=2
  2x : Gain  Gain=2
  Add : Sum  Inputs=-+
  Add1 : Sum
  Add2 : Sum  Inputs=-+
  Add3 : Sum  Inputs=+-
  Add4 : Sum
  Constant : Constant
  Constant10 : Constant  Value=0
  Constant4 : Constant
  Constant9 : Constant
  D : Constant  Value=10^(-8)
  Divide : Product  Inputs=*/
  Divide1 : Product  Inputs=**/
  Gain2 : Gain  Gain=0.5
  I-t : Scope
  Integrator : Integrator
  Integrator Initial condition source : Integrator  InitialConditionSource=external
  Math Function : Math  Operator=pow  SaturateOnIntegerOverflow=on
  Math Function1 : Math  Operator=square  SaturateOnIntegerOverflow=on
  Product1 : Product
  Product2 : Product
  Product3 : Product  Inputs=3
  Product4 : Product
  R_off : Constant  Value=20000
  R_on : Constant  Value=100
  R_on1 : Constant  Value=100
  Switch : Switch  Threshold=1
  Switch1 : Switch
  V-t : Scope
  p : Constant  Value=10
  x-t : Scope
  x0 : Constant  Value=0.7
  𝜇_𝑣 : Constant  Value=10^(-14)
  Out1 : Outport
  Out2 : Outport  Port=2
  wires:
  Constant9/1 -> Switch/1
  Switch/1 -> Switch1/2, Switch1/1
  R_on/1 -> Divide1/1
  Integrator Initial condition source/1 -> Switch/3, Switch/2, x-t/1
  Integrator/1 -> Divide/1, Product4/2
  2p/1 -> Math Function/2
  Divide/1 -> I-t/1, Product3/1
  Switch1/1 -> Product2/2, Add/1, 2x/1
  𝜇_𝑣/1 -> Divide1/2
  Gain2/1 -> Integrator/1
  Math Function/1 -> Add3/2
  Add/1 -> Product1/1
  R_on1/1 -> Product2/1
  Constant/1 -> Add/2
  p/1 -> 2p/1
  D/1 -> Math Function1/1
  Divide1/1 -> Product3/3
  2x/1 -> Add2/2
  Product1/1 -> Add1/2
  R_off/1 -> Product1/2
  Add2/1 -> Math Function/1
  Constant4/1 -> Add3/1, Add2/1
  Product4/1 -> Out1/1, Out2/1, V-t/1
  Product2/1 -> Add1/1
  x0/1 -> Integrator Initial condition source/2
  Constant10/1 -> Switch1/3
  Product3/1 -> Integrator Initial condition source/1
  Add1/1 -> Divide/2
  Add3/1 -> Product3/2
  Math Function1/1 -> Divide1/3
  " V"/1 -> Add4/2
  In1/1 -> Add4/1
  Add4/1 -> Product4/1, Gain2/1

== system memristors_LSTM/Subsystem/Memristor crossbar4/Subsystem14 ==
  note: Memristor
  note: k
  note: for I-V
  note: Rmem
  note: f(x)
  note: for x
  note: for processing
  In1 : Inport
  " V" : Sin  Frequency=0.5  SampleTime=0
  2p : Gain  Gain=2
  2x : Gain  Gain=2
  Add : Sum  Inputs=-+
  Add1 : Sum
  Add2 : Sum  Inputs=-+
  Add3 : Sum  Inputs=+-
  Add4 : Sum
  Constant : Constant
  Constant10 : Constant  Value=0
  Constant4 : Constant
  Constant9 : Constant
  D : Constant  Value=10^(-8)
  Divide : Product  Inputs=*/
  Divide1 : Product  Inputs=**/
  Gain2 : Gain  Gain=0.5
  I-t : Scope
  Integrator : Integrator
  Integrator Initial condition source : Integrator  InitialConditionSource=external
  Math Function : Math  Operator=pow  SaturateOnIntegerOverflow=on
  Math Function1 : Math  Operator=square  SaturateOnIntegerOverflow=on
  Product1 : Product
  Product2 : Product
  Product3 : Product  Inputs=3
  Product4 : Product
  R_off : Constant  Value=20000
  R_on : Constant  Value=100
  R_on1 : Constant  Value=100
  Switch : Switch  Threshold=1
  Switch1 : Switch
  V-t : Scope
  p : Constant  Value=10
  x-t : Scope
  x0 : Constant  Value=0.7
  𝜇_𝑣 : Constant  Value=10^(-14)
  Out2 : Outport
  wires:
  Constant9/1 -> Switch/1
  Switch/1 -> Switch1/2, Switch1/1
  R_on/1 -> Divide1/1
  Integrator Initial condition source/1 -> Switch/3, Switch/2, x-t/1
  Integrator/1 -> Divide/1, Product4/2
  2p/1 -> Math Function/2
  Divide/1 -> I-t/1, Product3/1
  Switch1/1 -> Product2/2, Add/1, 2x/1
  𝜇_𝑣/1 -> Divide1/2
  Gain2/1 -> Integrator/1
  Math Function/1 -> Add3/2
  Add/1 -> Product1/1
  R_on1/1 -> Product2/1
  Constant/1 -> Add/2
  p/1 -> 2p/1
  D/1 -> Math Function1/1
  Divide1/1 -> Product3/3
  2x/1 -> Add2/2
  Product1/1 -> Add1/2
  R_off/1 -> Product1/2
  Add2/1 -> Math Function/1
  Constant4/1 -> Add3/1, Add2/1
  Product4/1 -> Out2/1, V-t/1
  Product2/1 -> Add1/1
  x0/1 -> Integrator Initial condition source/2
  Constant10/1 -> Switch1/3
  Product3/1 -> Integrator Initial condition source/1
  Add1/1 -> Divide/2
  Add3/1 -> Product3/2
  Math Function1/1 -> Divide1/3
  " V"/1 -> Add4/2
  In1/1 -> Add4/1
  Add4/1 -> Product4/1, Gain2/1

== system memristors_LSTM/Subsystem/Memristor crossbar4/Subsystem15 ==
  note: Memristor
  note: k
  note: for I-V
  note: Rmem
  note: f(x)
  note: for x
  note: for processing
  " V" : Sin  Amplitude=0.1  Frequency=0.5  SampleTime=0
  2p : Gain  Gain=2
  2x : Gain  Gain=2
  Add : Sum  Inputs=-+
  Add1 : Sum
  Add2 : Sum  Inputs=-+
  Add3 : Sum  Inputs=+-
  Constant : Constant
  Constant10 : Constant  Value=0
  Constant4 : Constant
  Constant9 : Constant
  D : Constant  Value=10^(-8)
  Divide : Product  Inputs=*/
  Divide1 : Product  Inputs=**/
  Gain2 : Gain  Gain=0.5
  I-t : Scope
  Integrator : Integrator
  Integrator Initial condition source : Integrator  InitialConditionSource=external
  Math Function : Math  Operator=pow  SaturateOnIntegerOverflow=on
  Math Function1 : Math  Operator=square  SaturateOnIntegerOverflow=on
  Product1 : Product
  Product2 : Product
  Product3 : Product  Inputs=3
  Product4 : Product
  R_off : Constant  Value=20000
  R_on : Constant  Value=100
  R_on1 : Constant  Value=100
  Switch : Switch  Threshold=1
  Switch1 : Switch
  V-t : Scope
  p : Constant  Value=10
  x-t : Scope
  x0 : Constant  Value=0.7
  𝜇_𝑣 : Constant  Value=10^(-14)
  Out1 : Outport
  Out2 : Outport  Port=2
  wires:
  Constant9/1 -> Switch/1
  Switch/1 -> Switch1/2, Switch1/1
  R_on/1 -> Divide1/1
  Integrator Initial condition source/1 -> Switch/3, Switch/2, x-t/1
  Integrator/1 -> Divide/1, Product4/2
  2p/1 -> Math Function/2
  Divide/1 -> I-t/1, Product3/1
  Switch1/1 -> Product2/2, Add/1, 2x/1
  𝜇_𝑣/1 -> Divide1/2
  Gain2/1 -> Integrator/1
  Math Function/1 -> Add3/2
  Add/1 -> Product1/1
  R_on1/1 -> Product2/1
  Constant/1 -> Add/2
  p/1 -> 2p/1
  D/1 -> Math Function1/1
  Divide1/1 -> Product3/3
  2x/1 -> Add2/2
  Product1/1 -> Add1/2
  R_off/1 -> Product1/2
  Add2/1 -> Math Function/1
  Constant4/1 -> Add3/1, Add2/1
  Product4/1 -> Out1/1, Out2/1, V-t/1
  Product2/1 -> Add1/1
  x0/1 -> Integrator Initial condition source/2
  Constant10/1 -> Switch1/3
  Product3/1 -> Integrator Initial condition source/1
  Add1/1 -> Divide/2
  Add3/1 -> Product3/2
  Math Function1/1 -> Divide1/3
  " V"/1 -> Gain2/1, Product4/1

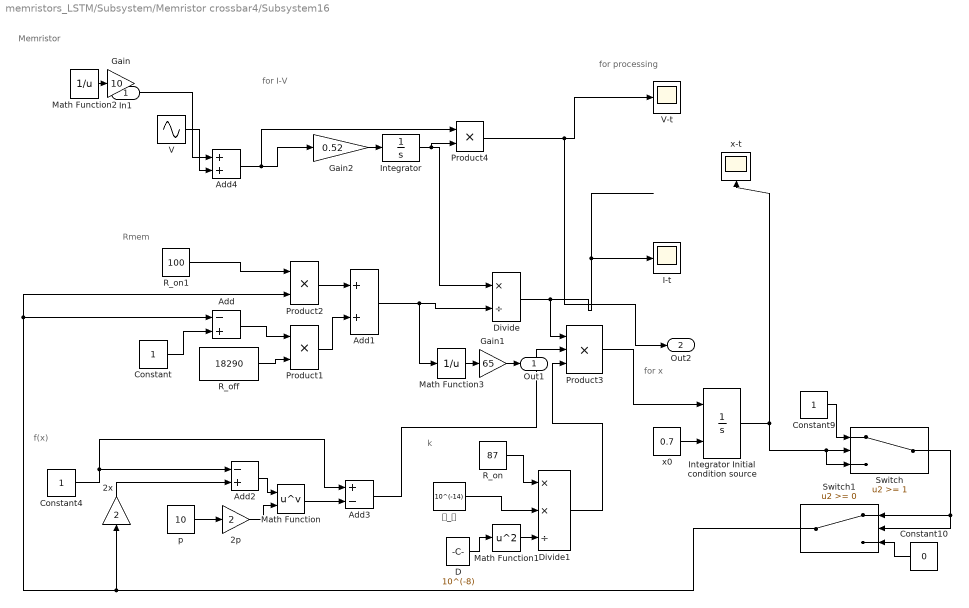
== system memristors_LSTM/Subsystem/Memristor crossbar4/Subsystem16 ==
  note: Memristor
  note: k
  note: for I-V
  note: Rmem
  note: f(x)
  note: for x
  note: for processing
  In1 : Inport
  " V" : Sin  Frequency=0.5  SampleTime=0
  2p : Gain  Gain=2
  2x : Gain  Gain=2
  Add : Sum  Inputs=-+
  Add1 : Sum
  Add2 : Sum  Inputs=-+
  Add3 : Sum  Inputs=+-
  Add4 : Sum
  Constant : Constant
  Constant10 : Constant  Value=0
  Constant4 : Constant
  Constant9 : Constant
  D : Constant  Value=10^(-8)
  Divide : Product  Inputs=*/
  Divide1 : Product  Inputs=**/
  Gain : Gain  Gain=10
  Gain1 : Gain  Gain=65
  Gain2 : Gain  Gain=0.52
  I-t : Scope
  Integrator : Integrator
  Integrator Initial condition source : Integrator  InitialConditionSource=external
  Math Function : Math  Operator=pow  SaturateOnIntegerOverflow=on
  Math Function1 : Math  Operator=square  SaturateOnIntegerOverflow=on
  Math Function2 : Math  Operator=reciprocal  SaturateOnIntegerOverflow=on
  Math Function3 : Math  Operator=reciprocal  SaturateOnIntegerOverflow=on
  Product1 : Product
  Product2 : Product
  Product3 : Product  Inputs=3
  Product4 : Product
  R_off : Constant  Value=18290
  R_on : Constant  Value=87
  R_on1 : Constant  Value=100
  Switch : Switch  Threshold=1
  Switch1 : Switch
  V-t : Scope
  p : Constant  Value=10
  x-t : Scope
  x0 : Constant  Value=0.7
  𝜇_𝑣 : Constant  Value=10^(-14)
  Out1 : Outport
  Out2 : Outport  Port=2
  wires:
  Constant9/1 -> Switch/1
  Switch/1 -> Switch1/2, Switch1/1
  R_on/1 -> Divide1/1
  Integrator Initial condition source/1 -> Switch/3, Switch/2, x-t/1
  2p/1 -> Math Function/2
  Divide/1 -> I-t/1, Product3/1
  Switch1/1 -> Product2/2, Add/1, 2x/1
  𝜇_𝑣/1 -> Divide1/2
  Gain2/1 -> Integrator/1
  Math Function/1 -> Add3/2
  Add/1 -> Product1/1
  R_on1/1 -> Product2/1
  Constant/1 -> Add/2
  p/1 -> 2p/1
  D/1 -> Math Function1/1
  Divide1/1 -> Product3/3
  2x/1 -> Add2/2
  Product1/1 -> Add1/2
  R_off/1 -> Product1/2
  Add2/1 -> Math Function/1
  Constant4/1 -> Add3/1, Add2/1
  Product4/1 -> Out2/1, V-t/1
  Product2/1 -> Add1/1
  x0/1 -> Integrator Initial condition source/2
  Constant10/1 -> Switch1/3
  Product3/1 -> Integrator Initial condition source/1
  Add3/1 -> Product3/2
  Math Function1/1 -> Divide1/3
  " V"/1 -> Add4/2
  In1/1 -> Add4/1
  Add4/1 -> Product4/1, Gain2/1
  Integrator/1 -> Divide/1, Product4/2
  Math Function2/1 -> Gain/1
  ? -> Math Function2/1
  Math Function3/1 -> Gain1/1
  Add1/1 -> Math Function3/1, Divide/2
  Gain1/1 -> Out1/1
